simulink model "ACDCMG_sim8"  (R2022a)
settings: Solver=FixedStepAuto  StartTime=0.0  StopTime=0.5  FixedStep=Ts  MaxStep=1e-2  RelTol=1e-3
InitFcn:
  | Set_parameters_R2018
undefined symbols (not defined in the file): D1, D_invs, dEgdT, Delta, dis11, dis12, dis2, dis3, dis4, dis5, dis6, DiscIntNeverNeededParam, EgRef, fn, Fnom, gcbh, H_invs, Ion, k1, Lithium, max_min, P_Load_3, P_nom_inv, Pnom_T1, Pnom_T2, Pnom_T3, Ql_Load_3, R_Load_9, R_Load_DC, Rl, Rls, Rsh_array5pc, sps_rtmsupport, Tref_K, Ts, Ts_Control, Ts_Inv, Ts_Power, Ts_PV, V1_LL_T3, Vmin_mppt, VnInv, Vnom_DC, Vnom_Diesel, Vnom_prim, Vnom_sec, Vnom_ter_AC_DC, VT_ref, Xl, Xls
libraries: spsCurrentMeasurementLib x40, spsRMSLib x29, spsSeriesRLCBranchLib x23, spsVoltageMeasurementLib x21, spsMeanLib x14, spsThreePhaseVIMeasurementLib x14, powerlib_extras x13, spsThreePhaseSeriesRLCBranchLib x12, spsBreakerLib x8, spsControlledVoltageSourceLib x8, spsPowerLib x8, spsControlledCurrentSourceLib x6
(part 3 of 11)

== system ACDCMG_sim8/PV Subsystem ==
  Bus Selector : BusSelector  OutputSignals=V_PV,I_PV  OutputAsBus=on
  Diode1 : spsDiodeLib/Diode  Ron=0.001  Lon=0  Vf=0.7  IC=0  UseSnubber=off  Rs=1e5  Cs=1e5  Measurements=on
  I : spsCurrentMeasurementLib/Current Measurement  PhasorSimulation=off  OutputType=Complex  PSBequivalent=0
  Ir1 : Constant  Value=1000
  PV Panel : Subsystem  AncestorBlock=spsPVArrayLib/PV Array  DialogController=POWERSYS.PowerSysDialog  LoadFcn=sps_rtmsupport('LoadFcn',gcbh);  StartFcn=sps_rtmsupport('StartFcn',gcbh);  StopFcn=sps_rtmsupport('StopFcn',gcbh);  mask(PV array){Npar=7, Nser=6, PlotType=one module @ 25 deg.C & specified irradiances, S_vec=1000, Temp_C_vec=[ 45 25  ], ModuleName=User-defined, PlotWhenSelected=off, Pm=250.205, Ncell=96, Voc=37.4, Isc=8.63, Vm=30.7, Im=8.15, beta_Voc_pc=-0.34, alpha_Isc_pc=0.05, beta_Voc=-0.12716, alpha_Isc=0.004315, IL=8.6686, I0=1.3965e-10, nI=0.6105, Rsh=311.9016, Rs=0.26776, RobustModel=off, RobustCellTemperature=313.3991, BAL=off, Tc=1e-6, Tfilter=0.0001}
      mask prompts: Npar "Parallel strings"; Nser "Series-connected modules per string"; S_vec "Irradiances (W/m2)"; Temp_C_vec "T_cell (deg. C)"; ModuleName "Module:"; PlotWhenSelected "Plot I-V and P-V characteristics when a module is selected"; Pm "Maximum Power (W)"; Ncell "Cells per module (Ncell)"; Voc "Open circuit voltage  Voc (V)"; Isc "Short-circuit current Isc (A)"; Vm "Voltage at maximum power point Vmp (V)"; Im "Current at maximum power point Imp (A)"; beta_Voc_pc "Temperature coefficient of Voc (%/deg.C)"; alpha_Isc_pc "Temperature coefficient of Isc (%/deg.C)"; beta_Voc "Temperature coefficient of Voc (V/deg.C)"; alpha_Isc "Temperature coefficient of Isc (A/deg.C)"; IL "Light-generated current IL (A)"; I0 "Diode saturation current I0 (A)"; nI "Diode ideality factor"; Rsh "Shunt resistance Rsh (ohms)"; Rs "Series resistance Rs (ohms)"; RobustModel "Robust discrete model"; RobustCellTemperature "Cell temperature, in deg.C. (input 2 is disabled)"; BAL "Break algebraic loop in internal model"; Tc "Break loop time constant (s)"; Tfilter "Measurement filter time constant (s)"
      mask help:
      | Implements a PV array built of strings of PV modules connected in parallel. Each string consists of modules connected in series.
      | Allows modeling of a variety of preset PV modules available from NREL System Advisor Model (Jan. 2014) as well as user-defined PV module.
      |
      | Input 1 = Sun irradiance, in W/m2, and input 2 = Cell temperature, in deg.C.
      mask init:
      | Block = gcb;
      | [k,k1,q,Tref_C,Tref_K,EgRef,dEgdT,Rsh_array5pc,VT_ref,Tsf,Tf,VIdiodePV,WantBlockChoice] = PVArrayInit(Block, Nser, Npar, Ncell, Rsh, nI, Tfilter, Voc, I0);
      | powericon('SetInternalModels','set',Block,WantBlockChoice);
      | sps_rtmsupport('parametereditingmodes',Block, [3 6 7 23]);
      settings: CopyFcn=sps_rtmsupport('CopyFcn',gcbh);  DeleteFcn=sps_rtmsupport('DeleteFcn',gcbh);  UndoDeleteFcn=sps_rtmsupport('UndoDeleteFcn',gcbh);  ModelCloseFcn=sps_rtmsupport('ModelCloseFcn',gcbh);  PreSaveFcn=sps_rtmsupport('PreSaveFcn',gcbh);  PostSaveFcn=sps_rtmsupport('PostSaveFcn',gcbh);  NameChangeFcn=sps_rtmsupport('NameChangeFcn',gcbh);  PreCopyFcn=sps_rtmsupport('PreCopyFcn',gcbh);  CloseFcn=sps_rtmsupport('CloseFcn',gcbh);  PreDeleteFcn=sps_rtmsupport('PreDeleteFcn',gcbh);
      settings: AttributesFormatString=|
      | %<ModuleName>
      | %<Nser>-module string
      | %<Npar> parallel strings
      settings: OpenFcn=|
      | %assignin('base','PVMaskOpening',1);
      | %open_system(gcb,'mask')
      | %assignin('base','PVMaskOpening',0);
      | sps_rtmsupport('OpenFcn',gcbh, [3 6 7 23]);
      mask Help: helpview(psbhelp);
      mask TypeOptions PlotType: one module @ 25 deg.C & specified irradiances | array @ 25 deg.C & specified irradiances | array @ 1000 W/m2 & specified temperatures
      mask Callback PlotType: PVArrayCback(gcb)
